simulink subsystem "Tester_SS"  (R2023b)
settings: Solver=VariableStepAuto  StartTime=0.0  StopTime=10.0  RelTol=1e-3
undefined symbols (not defined in the file or in its folder): canChannel
libraries: canlib x5, canmsglib x5
settings Model: Creator=nickj  LastModifiedBy=diego

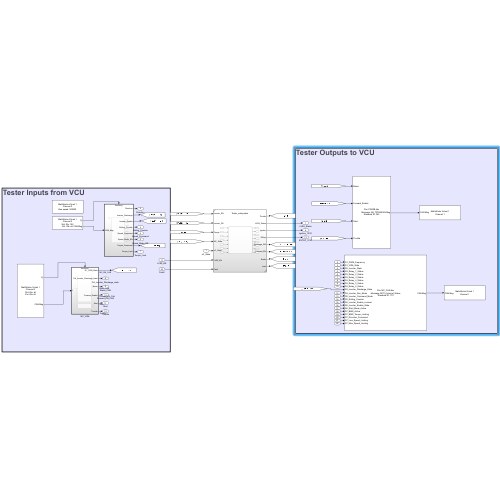
[thumbnail: Simulink's stored preview of the top-level diagram]
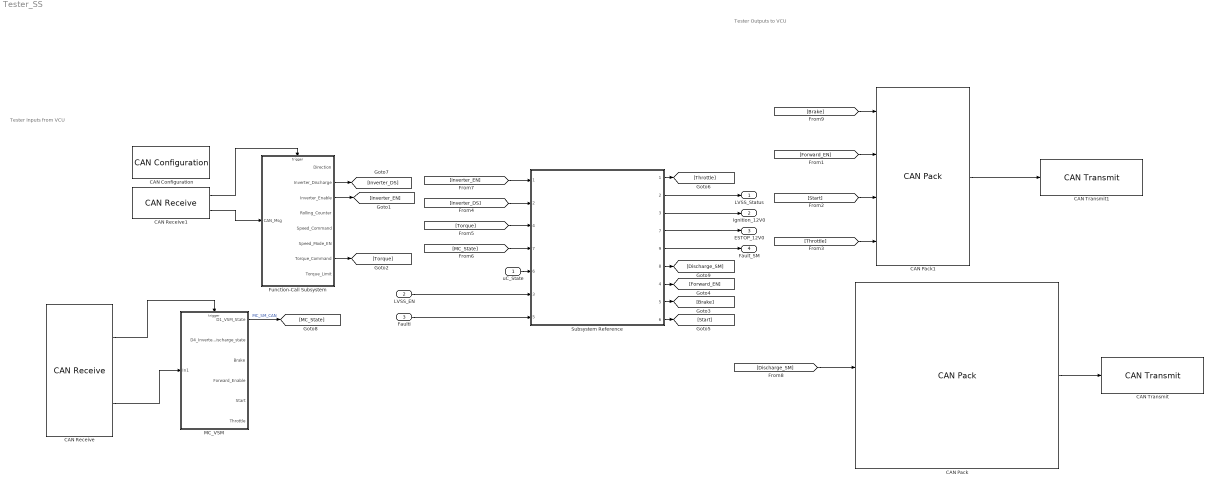
== system Tester_SS ==
  note: Tester Inputs from VCU
  note: Tester Outputs to VCU
  uC_State : Inport
  LVSS_EN : Inport  Port=2
  FaultI : Inport  Port=3
  CAN Configuration : canlib/CAN Configuration  BlockHandle=9543.0007  Device=MathWorks Virtual 1 (Channel 2)  DeviceMenu=MathWorks Virtual 1 (Channel 2)  ObjConstructor=canChannel('MathWorks', 'Virtual 1', 2)  BusSpeed=500000  EnableBitParameters=off  AckMode=Normal
  CAN Pack : canmsglib/CAN Pack  CANdbFile=C:\Users\heyka\MATLAB\Projects\VCU_C\MC_CAN.dbc  MsgList=M170_Internal_States  MsgName=M170_Internal_States  MsgIDType=Standard (11-bit identifier)  MsgIdentifier=170  MsgLength=8  Remote=off  ApplyMinMax=off  BusOutput=off  SignalInfo={'D1_PWM_Frequency','8','8','LE','unsigned','Standard','0','1','0','0','255';'D1_VSM_State','0','8','LE','unsigned','Standard','0','1','0','0','15';'D2_Inverter_State','16','8','LE','unsigned','Standard','0','1','0','0','255';'D3_Relay_1_Status','24','1','LE','unsigned','Standard','0','1','0','0','1';'D3_Relay_2_Status','25','1','LE','unsigned','Standard','0','1','0','0','1';'D3_Relay_3_Status','26','1','LE','unsigned','Standard','0','1','0','0','1';'D3_Relay_4_Status','27','1','LE','unsigned','Standard','0','1','0','0','1';'D3_Relay_5_Status','28','1','LE','unsigned','Standard','0','1','0','0','1';'D3_Relay_6_Status','29','1','LE','unsigned','Standard','0','1','0','0','1';'D4_Inverter_Discharge_State','37','3','LE','unsigned','Standard','0','1','0','0','7';'D4_Inverter_Run_Mode','32','1','LE','unsigned','Standard','0','1','0','0','1';'D5_Inverter_Command_Mode','40','1','LE','unsigned','Standard','0','1','0','0','1';'D5_Rolling_Counter','44','4','LE','unsigned','Standard','0','1','0','0','15';'D6_Inverter_Enable_Lockout','55','1','LE','unsigned','Standard','0','1','0','0','1';'D6_Inverter_Enable_State','48','1','LE','unsigned','Standard','0','1','0','0','1';'D6_Start_Mode_Active','54','1','LE','unsigned','Standard','0','1','0','0','1';'D7_BMS_Active','57','1','LE','unsigned','Standard','0','1','0','0','1';'D7_BMS_Torque_Limiting','58','1','LE','unsigned','Standard','0','1','0','0','1';'D7_Direction_Command','56','1','LE','unsigned','Standard','0','1','0','0','1';'D7_Low_Speed_Limiting','61','1','LE','unsigned','Standard','0','1','0','0','1';'D7_Max_Speed_Limiting','59','1','LE','unsigned','Standard','0','1','0','0','1'}
      settings: LibrarySourceBlock=canlib/CAN Pack  DataFormat=CANdb specified signals
  CAN Pack1 : canmsglib/CAN Pack  CANdbFile=C:\Users\heyka\MATLAB\Projects\VCU_C\PRJDB.dbc  MsgList=N8_TPDO0  MsgName=N8_TPDO0  MsgIDType=Standard (11-bit identifier)  MsgIdentifier=392  MsgLength=5  Remote=off  ApplyMinMax=off  BusOutput=off  SignalInfo={'Brake','1','16','LE','signed','Standard','0','1','0','0','494967295';'Forward_Enable','0','1','LE','unsigned','Standard','0','1','0','0','494967295';'Start','17','1','LE','unsigned','Standard','0','1','0','-Inf','Inf';'Throttle','18','16','LE','signed','Standard','0','1','0','-32768','32767'}
      settings: LibrarySourceBlock=canlib/CAN Pack  DataFormat=CANdb specified signals
  CAN Receive : canlib/CAN Receive  BlockHandle=9546.0007  Device=MathWorks Virtual 1 (Channel 2)  DeviceMenu=MathWorks Virtual 1 (Channel 2)  ObjConstructor=canChannel('MathWorks', 'Virtual 1', 2)  EnableStandardIDsFilter=off  StdIDsCombo=Allow all  StandardIDs=0  EnableExtendedIDsFilter=off  ExtIDsCombo=Allow all  ExtendedIDs=0  SampleTime=0.01  MsgsPerTimestep=all  InternalFilterUpdateStatus=on  BusOutput=off
  CAN Receive1 : canlib/CAN Receive  BlockHandle=9547.0007  Device=MathWorks Virtual 1 (Channel 2)  DeviceMenu=MathWorks Virtual 1 (Channel 2)  ObjConstructor=canChannel('MathWorks', 'Virtual 1', 2)  EnableStandardIDsFilter=off  StdIDsCombo=Allow only  StandardIDs=192  EnableExtendedIDsFilter=off  ExtIDsCombo=Allow all  ExtendedIDs=0  SampleTime=0.01  MsgsPerTimestep=all  InternalFilterUpdateStatus=on  BusOutput=off
  CAN Transmit : canlib/CAN Transmit  BlockHandle=9548.0007  Device=MathWorks Virtual 1 (Channel 1)  DeviceMenu=MathWorks Virtual 1 (Channel 1)  ObjConstructor=canChannel('MathWorks', 'Virtual 1', 1)  EnableEventTransmit=off  EnablePeriodicTransmit=off  MessagePeriod=1.000
  CAN Transmit1 : canlib/CAN Transmit  BlockHandle=9549.0007  Device=MathWorks Virtual 1 (Channel 1)  DeviceMenu=MathWorks Virtual 1 (Channel 1)  ObjConstructor=canChannel('MathWorks', 'Virtual 1', 1)  EnableEventTransmit=off  EnablePeriodicTransmit=off  MessagePeriod=1.000
  Function-Call Subsystem : Subsystem  TreatAsAtomicUnit=on
  MC_VSM : Subsystem  TreatAsAtomicUnit=on
  Subsystem Reference : Subsystem  ReferencedSubsystem=Tester_subsystem
      settings: PortSchema="{\"entries\":[{\"content\":{\"sides\":[{\"content\":{\"connectorIds\":[\"In1\",\"In2\",\"In4\",\"In7\",\"In6\",\"In3\",\"In5\"]},\"type\":\"ConnectorPlacement.EquallySpacedRectSide\",\"uuid\":\"dc30693d-6009-44ff-85e6-3f077094237c\"},{\"content\":{\"connectorIds\":[\"Out1\",\"Out2\",\"Out3\",\"Out7\",\"Out9\",\"Out8\",\"Out4\",\"Out5\",\"Out6\"],\"side\":\"RIGHT\"},\"type\":\"ConnectorPlacement.EquallySpacedRectSide\",\"uuid\":\"fb134251-bbd7-4a8f-a3d6-711305ba7863\"},{\"content\":{\"side\":\"TOP\"},\"type\":\"ConnectorPlacement.EquallySpacedRectSide\",\"uuid\":\"adf826c5-77bc-492b-9a9e-2ecad5d2f2a1\"}]},\"type\":\"ConnectorPlacement.EquallySpacedConnector\",\"uuid\":\"5d05b1d4-b527-468d-9dd4-c848a0c99d01\"}],\"packageUris\":[\"http://schema.mathworks.com/mf0/Connector/R2020b\"],\"version\":\"1.0\"}"
  LVSS_Status : Outport
  Ignition_12V0 : Outport  Port=2
  ESTOP_12V0 : Outport  Port=3
  Fault_SM : Outport  Port=4
  wires:
  [Start] -> CAN Pack1/3
  MC_VSM/1(D1_VSM_State) -> [MC_State]  "MC_SM_CAN"
  Subsystem Reference/3 -> Ignition_12V0/1
  Subsystem Reference/6 -> [Start]
  uC_State/1 -> Subsystem Reference/6
  [MC_State] -> Subsystem Reference/7
  CAN Receive/2 -> MC_VSM/1(In1)
  [Discharge_SM] -> CAN Pack/10
  Function-Call Subsystem/7(Torque_Command) -> [Torque]
  [Torque] -> Subsystem Reference/4
  CAN Pack1/1 -> CAN Transmit1/1
  CAN Receive1/1 -> Function-Call Subsystem/Trigger
  Function-Call Subsystem/2(Inverter_Discharge) -> [Inverter_DS]
  CAN Pack/1 -> CAN Transmit/1
  [Brake] -> CAN Pack1/1
  Function-Call Subsystem/3(Inverter_Enable) -> [Inverter_EN]
  FaultI/1 -> Subsystem Reference/5
  Subsystem Reference/2 -> LVSS_Status/1
  CAN Receive/1 -> MC_VSM/Trigger
  Subsystem Reference/7 -> ESTOP_12V0/1
  [Forward_EN] -> CAN Pack1/2
  [Inverter_EN] -> Subsystem Reference/1
  Subsystem Reference/4 -> [Forward_EN]
  LVSS_EN/1 -> Subsystem Reference/3
  Subsystem Reference/8 -> [Discharge_SM]
  [Inverter_DS] -> Subsystem Reference/2
  [Throttle] -> CAN Pack1/4
  Subsystem Reference/1 -> [Throttle]
  Subsystem Reference/5 -> [Brake]
  CAN Receive1/2 -> Function-Call Subsystem/1(CAN_Msg)
  Subsystem Reference/9 -> Fault_SM/1

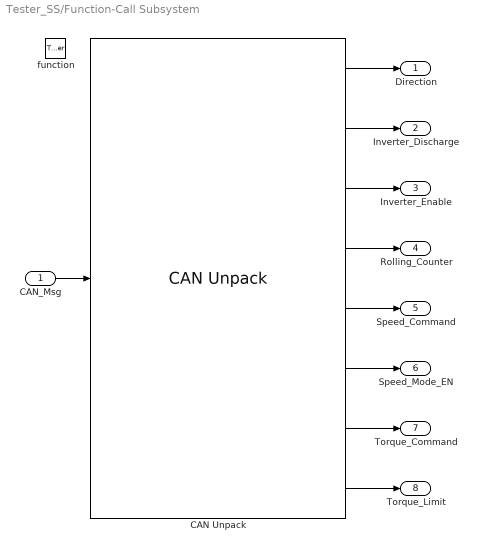
== system Tester_SS/Function-Call Subsystem ==
  CAN_Msg : Inport
  function : TriggerPort  TriggerType=function-call  VariantControl=(inherit)
  CAN Unpack : canmsglib/CAN Unpack  CANdbFile=C:\Users\heyka\MATLAB\Projects\VCU_C\MC_CAN.dbc  MsgList=M192_Command_Message  MsgName=M192_Command_Message  MsgIDType=Standard (11-bit identifier)  MsgIdentifier=192  MsgLength=8  SignalInfo={'Direction_Command','32','1','LE','unsigned','Standard','0','1','0','0','1';'Inverter_Discharge','41','1','LE','unsigned','Standard','0','1','0','0','1';'Inverter_Enable','40','1','LE','unsigned','Standard','0','1','0','0','1';'RollingCounter','44','4','LE','unsigned','Standard','0','1','0','0','15';'Speed_Command','16','16','LE','signed','Standard','0','1','0','-32768','32767';'Speed_Mode_Enable','42','1','LE','unsigned','Standard','0','1','0','0','1';'Torque_Command','0','16','LE','signed','Standard','0','0.1','0','-3276.8','3276.7';'Torque_Limit_Command','48','16','LE','signed','Standard','0','0.1','0','-3276.8','3276.7'}  IDPort=off  TimestampPort=off  ErrorPort=off  RemotePort=off  LengthPort=off  StatusPort=off  ApplyMinMax=off
      settings: DataFormat=CANdb specified signals
  Direction : Outport
  Inverter_Discharge : Outport  Port=2
  Inverter_Enable : Outport  Port=3
  Rolling_Counter : Outport  Port=4
  Speed_Command : Outport  Port=5
  Speed_Mode_EN : Outport  Port=6
  Torque_Command : Outport  Port=7
  Torque_Limit : Outport  Port=8
  wires:
  CAN Unpack/1 -> Direction/1
  CAN_Msg/1 -> CAN Unpack/1
  CAN Unpack/2 -> Inverter_Discharge/1
  CAN Unpack/4 -> Rolling_Counter/1
  CAN Unpack/3 -> Inverter_Enable/1
  CAN Unpack/5 -> Speed_Command/1
  CAN Unpack/6 -> Speed_Mode_EN/1
  CAN Unpack/7 -> Torque_Command/1
  CAN Unpack/8 -> Torque_Limit/1

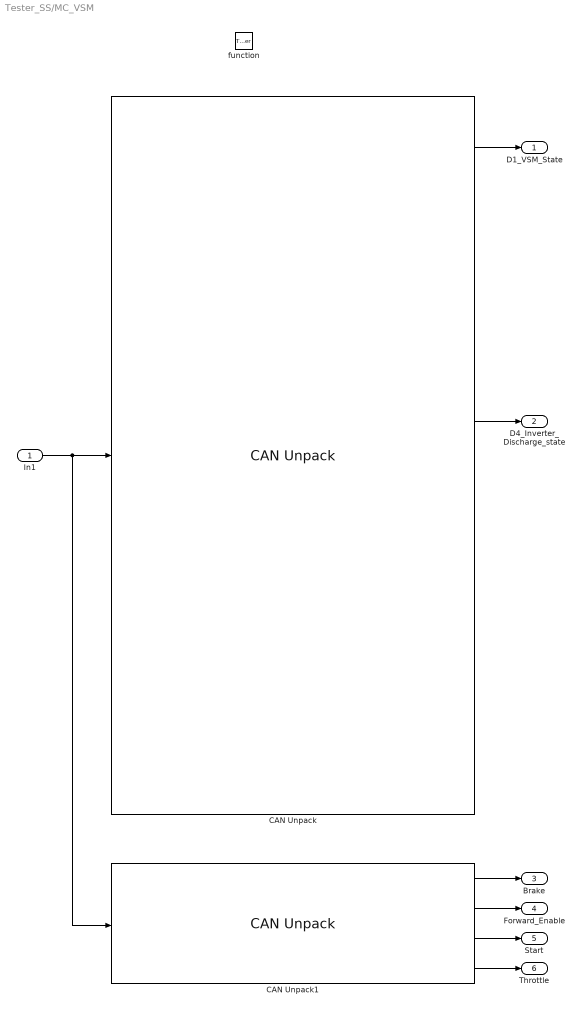
== system Tester_SS/MC_VSM ==
  In1 : Inport
  function : TriggerPort  TriggerType=function-call  VariantControl=(inherit)
  CAN Unpack : canmsglib/CAN Unpack  CANdbFile=C:\Users\heyka\MATLAB\Projects\VCU_C\MC_CAN.dbc  MsgList=M170_Internal_States  MsgName=M170_Internal_States  MsgIDType=Standard (11-bit identifier)  MsgIdentifier=170  MsgLength=8  SignalInfo={'D1_PWM_Frequency','8','8','LE','unsigned','Standard','0','1','0','0','255';'D1_VSM_State','0','8','LE','unsigned','Standard','0','1','0','0','15';'D2_Inverter_State','16','8','LE','unsigned','Standard','0','1','0','0','255';'D3_Relay_1_Status','24','1','LE','unsigned','Standard','0','1','0','0','1';'D3_Relay_2_Status','25','1','LE','unsigned','Standard','0','1','0','0','1';'D3_Relay_3_Status','26','1','LE','unsigned','Standard','0','1','0','0','1';'D3_Relay_4_Status','27','1','LE','unsigned','Standard','0','1','0','0','1';'D3_Relay_5_Status','28','1','LE','unsigned','Standard','0','1','0','0','1';'D3_Relay_6_Status','29','1','LE','unsigned','Standard','0','1','0','0','1';'D4_Inverter_Discharge_State','37','3','LE','unsigned','Standard','0','1','0','0','7';'D4_Inverter_Run_Mode','32','1','LE','unsigned','Standard','0','1','0','0','1';'D5_Inverter_Command_Mode','40','1','LE','unsigned','Standard','0','1','0','0','1';'D5_Rolling_Counter','44','4','LE','unsigned','Standard','0','1','0','0','15';'D6_Inverter_Enable_Lockout','55','1','LE','unsigned','Standard','0','1','0','0','1';'D6_Inverter_Enable_State','48','1','LE','unsigned','Standard','0','1','0','0','1';'D6_Start_Mode_Active','54','1','LE','unsigned','Standard','0','1','0','0','1';'D7_BMS_Active','57','1','LE','unsigned','Standard','0','1','0','0','1';'D7_BMS_Torque_Limiting','58','1','LE','unsigned','Standard','0','1','0','0','1';'D7_Direction_Command','56','1','LE','unsigned','Standard','0','1','0','0','1';'D7_Low_Speed_Limiting','61','1','LE','unsigned','Standard','0','1','0','0','1';'D7_Max_Speed_Limiting','59','1','LE','unsigned','Standard','0','1','0','0','1'}  IDPort=off  TimestampPort=off  ErrorPort=off  RemotePort=off  LengthPort=off  StatusPort=off  ApplyMinMax=off
      settings: LibrarySourceBlock=canlib/CAN Unpack  DataFormat=CANdb specified signals
  CAN Unpack1 : canmsglib/CAN Unpack  CANdbFile=C:\Users\heyka\MATLAB\Projects\VCU_C\PRJDB.dbc  MsgList=N8_TPDO0  MsgName=N8_TPDO0  MsgIDType=Standard (11-bit identifier)  MsgIdentifier=392  MsgLength=5  SignalInfo={'Brake','1','16','LE','signed','Standard','0','1','0','0','494967295';'Forward_Enable','0','1','LE','unsigned','Standard','0','1','0','0','494967295';'Start','17','1','LE','unsigned','Standard','0','1','0','-Inf','Inf';'Throttle','18','16','LE','signed','Standard','0','1','0','-32768','32767'}  IDPort=off  TimestampPort=off  ErrorPort=off  RemotePort=off  LengthPort=off  StatusPort=off  ApplyMinMax=off
      settings: LibrarySourceBlock=canlib/CAN Unpack  DataFormat=CANdb specified signals
  D1_VSM_State : Outport
  D4_Inverter_Discharge_state : Outport  Port=2
  Brake : Outport  Port=3  OutDataTypeStr=int32
  Forward_Enable : Outport  Port=4  OutDataTypeStr=uint32
  Start : Outport  Port=5  OutDataTypeStr=uint32
  Throttle : Outport  Port=6  OutDataTypeStr=int32
  wires:
  CAN Unpack1/4 -> Throttle/1
  CAN Unpack1/3 -> Start/1
  CAN Unpack1/2 -> Forward_Enable/1
  CAN Unpack1/1 -> Brake/1
  CAN Unpack/10 -> D4_Inverter_Discharge_state/1
  CAN Unpack/2 -> D1_VSM_State/1
  In1/1 -> CAN Unpack/1, CAN Unpack1/1
